simulink model "SIFT"  (R2016a)
settings: Solver=FixedStepDiscrete  SolverMode=SingleTasking  StartTime=0  StopTime=5  RelTol=1e-3
undefined symbols (not defined in the file): gray, Rec, SDTV
libraries: visionhdlfilter x4, hdlsllib x3, visionhdlio x2, visionconversions x1, visionsources x1, visiongeotforms x1
settings Model: Creator=Gururaja  LastModifiedBy=Gururaja
settings OptimizationCC: BlockReduction=off  ConditionallyExecuteInputs=off  DefaultParameterBehavior=Inlined
settings DebuggingCC: AlgebraicLoopMsg=error  SingleTaskRateTransMsg=error  ParameterPrecisionLossMsg=none  IntegerSaturationMsg=none
settings HardwareCC: ProdBitPerPointer=32  ProdLargestAtomicFloat=None  ProdIntDivRoundTo=Undefined  ProdEndianess=Unspecified  ProdWordSize=32  ProdHWDeviceType=ASIC/FPGA->ASIC/FPGA  ProdEqTarget=off

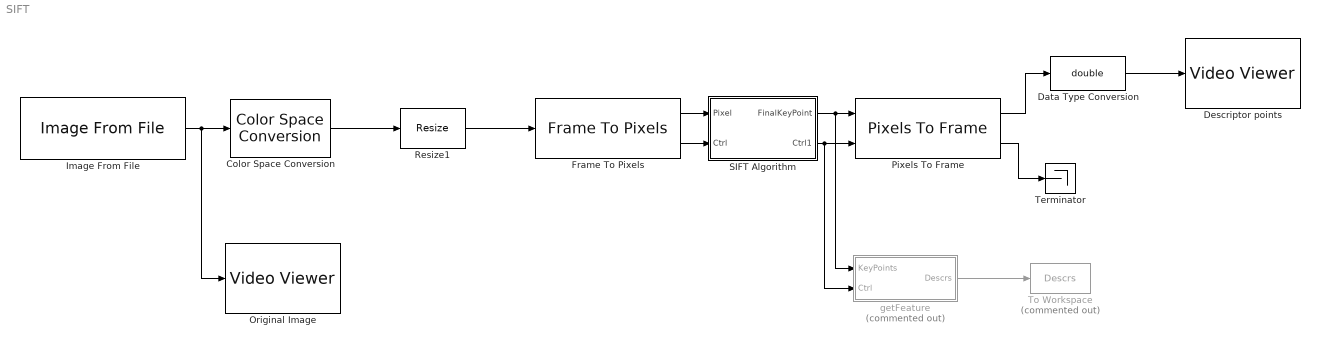
== system SIFT ==
  Color Space Conversion : visionconversions/Color Space  Conversion  conversion=Obsolete  conversionActive=R'G'B' to intensity  wp_str=D65  rec=Rec. 601 (SDTV)  sys=1125/60/2:1  imagePorts=One multidimensional signal
  Data Type Conversion : DataTypeConversion  OutDataTypeStr=double
  Descriptor points : VideoViewer  colormapValue=gray(256)  FigPos=[1 822 1536 724]
  Frame To Pixels : visionhdlio/Frame To Pixels  NumComponents=1  VideoFormat=240p  ActivePixelsPerLine=32  ActiveVideoLines=18  TotalPixelsPerLine=42  TotalVideoLines=28  StartingActiveLine=6  FrontPorch=5  SampleTime=0
  Image From File : visionsources/Image From File  Tag=vipblks_nd  FileName=E:\PROJECTS\FINAL YEAR PROJECT\ATTEMPTS\WORKING\SIFT-Scale-Invariant-Feature-Transform\lenatrain.jpg  imagePorts=One multidimensional signal  Ts=1  ImageDataType=Inherit from input image  Signed=off  WordLength=32  sdImageDataType=uint(8)  FractionLengthMode=Best precision  FractionLength=10  OutPortLabels=R|G|B
  Original Image : VideoViewer  colormapValue=gray(256)  FigPos=[1 822 1536 724]
  Pixels To Frame : visionhdlio/Pixels To Frame  NumComponents=1  VideoFormat=240p  ActivePixelsPerLine=32  ActiveVideoLines=18  TotalPixelsPerLine=42  TotalVideoLines=28
  Resize1 : visiongeotforms/Resize  specify=Number of output rows and columns  rfactor=[200 150]  outCols=25  outRows=25  outRowsCols=[240 320]  interp_method=Bilinear  antialias=on  useROI=off  roiFlag=off  prodOutputMode=Binary point scaling  prodOutputWordLength=32  prodOutputFracLength=10  roundingMode=Nearest  overflowMode=on
  SIFT Algorithm : Subsystem
  Terminator : Terminator
  To Workspace : ToWorkspace  Commented=on  VariableName=Descrs  SaveFormat=Timeseries  SampleTime=-1
  getFeature : Subsystem  Commented=on
  wires:
  Resize1/1 -> Frame To Pixels/1
  Frame To Pixels/1 -> SIFT Algorithm/1(Pixel)
  Frame To Pixels/2 -> SIFT Algorithm/2(Ctrl)
  SIFT Algorithm/1(FinalKeyPoint) -> getFeature/1(KeyPoints), Pixels To Frame/1
  SIFT Algorithm/2(Ctrl1) -> getFeature/2(Ctrl), Pixels To Frame/2
  Pixels To Frame/2 -> Terminator/1
  Pixels To Frame/1 -> Data Type Conversion/1
  Data Type Conversion/1 -> Descriptor points/1
  getFeature/1(Descrs) -> To Workspace/1
  Image From File/1 -> Original Image/1, Color Space Conversion/1
  Color Space Conversion/1 -> Resize1/1

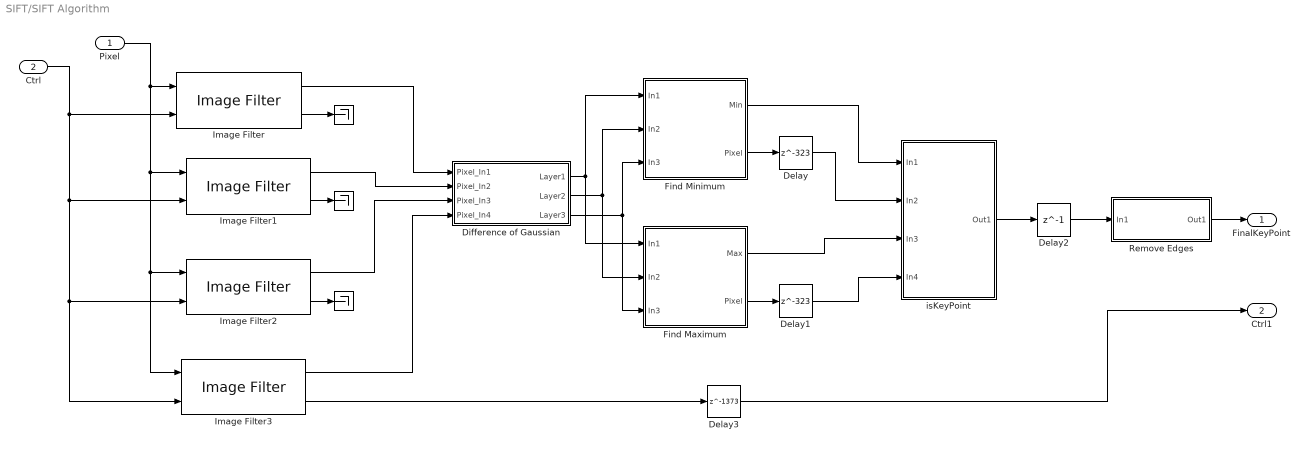
== system SIFT/SIFT Algorithm ==
  Pixel : Inport
  Ctrl : Inport  Port=2
  " " : Terminator
  " " : Terminator
  " " : Terminator
  Delay : Delay  DelayLength=323  InitialCondition=0
  Delay1 : Delay  DelayLength=323  InitialCondition=0
  Delay2 : Delay  DelayLength=1  InitialCondition=0
  Delay3 : Delay  DelayLength=1373  InitialCondition=0
  Difference of Gaussian : Subsystem
  Find Maximum : Subsystem
  Find Minimum : Subsystem
  Image Filter{,1..3} (4 alike) : visionhdlfilter/Image Filter  Coefficients=[ 1, 0; 0, -1 ]  PaddingMethod=Constant  PaddingValue=0  LineBufferSize=2048  roundingMode=Floor  overflowMode=off  CoeffMin=[]  CoeffMax=[]  OutputMin=[]  OutputMax=[]  SimulateUsing=Code generation
  Remove Edges : Subsystem
  isKeyPoint : Subsystem
  FinalKeyPoint : Outport
  Ctrl1 : Outport  Port=2
  wires:
  Pixel/1 -> Image Filter/1, Image Filter1/1, Image Filter3/1, Image Filter2/1
  Ctrl/1 -> Image Filter/2, Image Filter1/2, Image Filter2/2, Image Filter3/2
  Image Filter2/2 -> " "/1
  Image Filter1/2 -> " "/1
  Image Filter/2 -> " "/1
  Image Filter/1 -> Difference of Gaussian/1(Pixel_In1)
  Image Filter1/1 -> Difference of Gaussian/2(Pixel_In2)
  Image Filter2/1 -> Difference of Gaussian/3(Pixel_In3)
  Image Filter3/1 -> Difference of Gaussian/4(Pixel_In4)
  Difference of Gaussian/1(Layer1) -> Find Maximum/1(In1), Find Minimum/1(In1)
  Difference of Gaussian/2(Layer2) -> Find Maximum/2(In2), Find Minimum/2(In2)
  Difference of Gaussian/3(Layer3) -> Find Maximum/3(In3), Find Minimum/3(In3)
  Find Minimum/2(Pixel) -> Delay/1
  Find Minimum/1(Min) -> isKeyPoint/1(In1)
  Delay/1 -> isKeyPoint/2(In2)
  Delay1/1 -> isKeyPoint/4(In4)
  isKeyPoint/1(Out1) -> Delay2/1
  Delay2/1 -> Remove Edges/1(In1)
  Remove Edges/1(Out1) -> FinalKeyPoint/1
  Image Filter3/2 -> Delay3/1
  Delay3/1 -> Ctrl1/1
  Find Maximum/1(Max) -> isKeyPoint/3(In3)
  Find Maximum/2(Pixel) -> Delay1/1

== system SIFT/getFeature ==
  KeyPoints : Inport
  Ctrl : Inport  Port=2
  Delay : Delay  DelayLength=647  InitialCondition=0
  Delay1 : Delay  DelayLength=647  InitialCondition=0
  Descriptor : Subsystem
  HDL FIFO : hdlsllib/HDL Operations/HDL FIFO  fifo_size=1000  ratio=1  push_msg=Warning  pop_msg=Warning  show_empty=on  show_full=on  show_num=on
  MATLAB Function : MATLAB Function  TreatAsAtomicUnit=on
  MagORI : Subsystem
  Terminator : Terminator
  Terminator1 : Terminator
  Descrs : Outport
  wires:
  KeyPoints/1 -> HDL FIFO/1, Delay/1
  Delay/1 -> MagORI/1(Pixel)
  Ctrl/1 -> HDL FIFO/2, Delay1/1
  Delay1/1 -> MagORI/2(Ctrl)
  HDL FIFO/4 -> Terminator/1
  HDL FIFO/3 -> Terminator1/1
  MagORI/1(Mag) -> Descriptor/1(In1)
  HDL FIFO/2 -> MATLAB Function/3(empty)
  Descriptor/1(KeyPoint) -> MATLAB Function/2(KPdis)
  HDL FIFO/1 -> MATLAB Function/1(KPsource)
  Descriptor/2(Desc) -> MATLAB Function/4(descr)
  MATLAB Function/2(descrs) -> Descrs/1
  MATLAB Function/1(y) -> HDL FIFO/3

== system SIFT/SIFT Algorithm/Difference of Gaussian ==
  Pixel_In1 : Inport
  Pixel_In2 : Inport  Port=2
  Pixel_In3 : Inport  Port=3
  Pixel_In4 : Inport  Port=4
  Delay : Delay  DelayLength=13  InitialCondition=0
  Delay1 : Delay  DelayLength=1  InitialCondition=0
  Delay2 : Delay  DelayLength=1  InitialCondition=0
  Delay3 : Delay  DelayLength=12  InitialCondition=0
  Sum1 : Sum  Inputs=+-
  Sum2 : Sum  Inputs=+-
  Sum3 : Sum  Inputs=+-
  Layer1 : Outport
  Layer2 : Outport  Port=2
  Layer3 : Outport  Port=3
  wires:
  Pixel_In1/1 -> Sum3/1
  Pixel_In2/1 -> Sum3/2, Delay3/1
  Delay3/1 -> Sum1/1
  Pixel_In3/1 -> Sum2/1, Sum1/2
  Pixel_In4/1 -> Sum2/2
  Sum3/1 -> Delay/1
  Sum1/1 -> Delay1/1
  Sum2/1 -> Delay2/1
  Delay2/1 -> Layer3/1
  Delay1/1 -> Layer2/1
  Delay/1 -> Layer1/1

== system SIFT/SIFT Algorithm/Find Maximum ==
  In1 : Inport
  In2 : Inport  Port=2
  In3 : Inport  Port=3
  Min/Max DOG1 : Subsystem
  Min/Max DOG2 : Subsystem
  Min/Max DOG3 : Subsystem
  MinMax : MinMax  Function=max  Inputs=26
  Max : Outport
  Pixel : Outport  Port=2
  wires:
  In2/1 -> Min/Max DOG1/1(In1)
  Min/Max DOG1/5(Out5) -> Pixel/1
  Min/Max DOG2/1(Out1) -> MinMax/18
  Min/Max DOG2/9(Out9) -> MinMax/26
  Min/Max DOG2/2(Out2) -> MinMax/19
  Min/Max DOG2/3(Out3) -> MinMax/20
  Min/Max DOG2/4(Out4) -> MinMax/21
  Min/Max DOG2/5(Out5) -> MinMax/22
  Min/Max DOG2/6(Out6) -> MinMax/23
  Min/Max DOG2/7(Out7) -> MinMax/24
  Min/Max DOG2/8(Out8) -> MinMax/25
  Min/Max DOG3/1(Out1) -> MinMax/1
  Min/Max DOG3/3(Out3) -> MinMax/3
  Min/Max DOG3/2(Out2) -> MinMax/2
  Min/Max DOG3/4(Out4) -> MinMax/4
  Min/Max DOG3/5(Out5) -> MinMax/5
  Min/Max DOG3/6(Out6) -> MinMax/6
  Min/Max DOG3/7(Out7) -> MinMax/7
  Min/Max DOG3/8(Out8) -> MinMax/8
  Min/Max DOG3/9(Out9) -> MinMax/9
  MinMax/1 -> Max/1
  Min/Max DOG1/1(Out1) -> MinMax/10
  Min/Max DOG1/2(Out2) -> MinMax/11
  Min/Max DOG1/3(Out3) -> MinMax/12
  Min/Max DOG1/4(Out4) -> MinMax/13
  Min/Max DOG1/6(Out6) -> MinMax/14
  Min/Max DOG1/7(Out7) -> MinMax/15
  Min/Max DOG1/8(Out8) -> MinMax/16
  Min/Max DOG1/9(Out9) -> MinMax/17
  In1/1 -> Min/Max DOG3/1(In1)
  In3/1 -> Min/Max DOG2/1(In1)

== system SIFT/SIFT Algorithm/Find Minimum ==
  In1 : Inport
  In2 : Inport  Port=2
  In3 : Inport  Port=3
  Min/Max DOG1 : Subsystem
  Min/Max DOG2 : Subsystem
  Min/Max DOG3 : Subsystem
  MinMax : MinMax  Inputs=26
  Min : Outport
  Pixel : Outport  Port=2
  wires:
  In2/1 -> Min/Max DOG1/1(In1)
  Min/Max DOG1/5(Out5) -> Pixel/1
  Min/Max DOG2/1(Out1) -> MinMax/18
  Min/Max DOG2/9(Out9) -> MinMax/26
  Min/Max DOG2/2(Out2) -> MinMax/19
  Min/Max DOG2/3(Out3) -> MinMax/20
  Min/Max DOG2/4(Out4) -> MinMax/21
  Min/Max DOG2/5(Out5) -> MinMax/22
  Min/Max DOG2/6(Out6) -> MinMax/23
  Min/Max DOG2/7(Out7) -> MinMax/24
  Min/Max DOG2/8(Out8) -> MinMax/25
  Min/Max DOG3/1(Out1) -> MinMax/1
  Min/Max DOG3/3(Out3) -> MinMax/3
  Min/Max DOG3/2(Out2) -> MinMax/2
  Min/Max DOG3/4(Out4) -> MinMax/4
  Min/Max DOG3/5(Out5) -> MinMax/5
  Min/Max DOG3/6(Out6) -> MinMax/6
  Min/Max DOG3/7(Out7) -> MinMax/7
  Min/Max DOG3/8(Out8) -> MinMax/8
  Min/Max DOG3/9(Out9) -> MinMax/9
  MinMax/1 -> Min/1
  Min/Max DOG1/1(Out1) -> MinMax/10
  Min/Max DOG1/2(Out2) -> MinMax/11
  Min/Max DOG1/3(Out3) -> MinMax/12
  Min/Max DOG1/4(Out4) -> MinMax/13
  Min/Max DOG1/6(Out6) -> MinMax/14
  Min/Max DOG1/7(Out7) -> MinMax/15
  Min/Max DOG1/8(Out8) -> MinMax/16
  Min/Max DOG1/9(Out9) -> MinMax/17
  In1/1 -> Min/Max DOG3/1(In1)
  In3/1 -> Min/Max DOG2/1(In1)

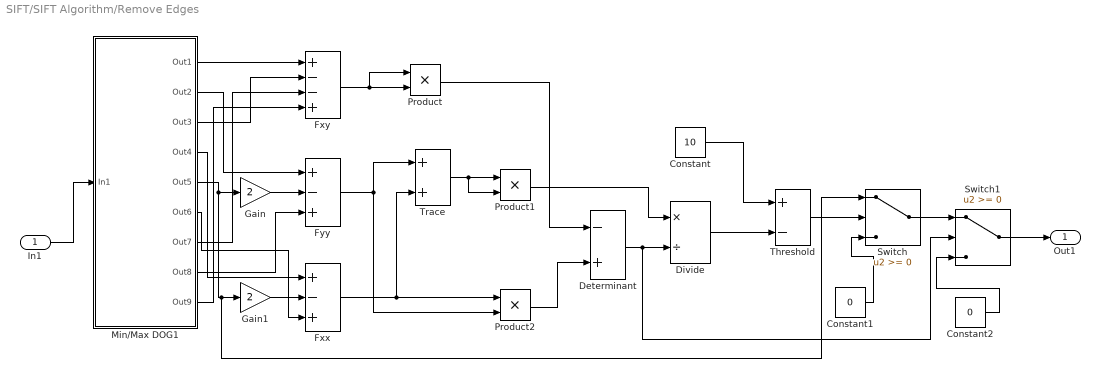
== system SIFT/SIFT Algorithm/Remove Edges ==
  In1 : Inport
  Constant : Constant  Value=10
  Constant1 : Constant  Value=0
  Constant2 : Constant  Value=0
  Determinant : Sum  Inputs=-+
  Divide : Product  Inputs=*/  SaturateOnIntegerOverflow=on
  Fxx : Sum  Inputs=+-+
  Fxy : Sum  Inputs=+--+
  Fyy : Sum  Inputs=+-+
  Gain : Gain  Gain=2
  Gain1 : Gain  Gain=2
  Min/Max DOG1 : Subsystem
  Product : Product
  Product1 : Product
  Product2 : Product
  Switch : Switch
  Switch1 : Switch
  Threshold : Sum  Inputs=+-
  Trace : Sum
  Out1 : Outport
  wires:
  In1/1 -> Min/Max DOG1/1(In1)
  Min/Max DOG1/1(Out1) -> Fxy/1
  Min/Max DOG1/3(Out3) -> Fxy/2
  Gain1/1 -> Fxx/2
  Gain/1 -> Fyy/2
  Min/Max DOG1/2(Out2) -> Fyy/1
  Min/Max DOG1/4(Out4) -> Fxx/1
  Min/Max DOG1/6(Out6) -> Fxx/3
  Min/Max DOG1/7(Out7) -> Fxy/3
  Min/Max DOG1/8(Out8) -> Fyy/3
  Min/Max DOG1/9(Out9) -> Fxy/4
  Fyy/1 -> Product2/2, Trace/1
  Fxy/1 -> Product/1, Product/2
  Trace/1 -> Product1/2, Product1/1
  Fxx/1 -> Trace/2, Product2/1
  Product2/1 -> Determinant/2
  Product/1 -> Determinant/1
  Determinant/1 -> Switch1/2, Divide/2
  Product1/1 -> Divide/1
  Divide/1 -> Threshold/2
  Constant/1 -> Threshold/1
  Threshold/1 -> Switch/2
  Constant1/1 -> Switch/3
  Min/Max DOG1/5(Out5) -> Switch/1, Gain1/1, Gain/1
  Switch/1 -> Switch1/1
  Constant2/1 -> Switch1/3
  Switch1/1 -> Out1/1

== system SIFT/SIFT Algorithm/isKeyPoint ==
  In1 : Inport
  In2 : Inport  Port=2
  In3 : Inport  Port=3
  In4 : Inport  Port=4
  " " : Constant  Value=0
  " " : Constant  Value=0
  Logical Operator : Logic  Operator=OR  AllPortsSameDT=off  OutDataTypeStr=boolean
  MinMax : MinMax  Function=max  Inputs=2
  Product : Product
  Product1 : Product
  Sum1 : Sum  Inputs=+-
  Sum2 : Sum  Inputs=+-
  Switch1 : Switch
  Switch2 : Switch
  Out1 : Outport
  wires:
  In1/1 -> Sum2/1
  In2/1 -> Sum2/2, Switch2/1, Product1/1
  Sum1/1 -> Switch1/2
  Sum2/1 -> Switch2/2
  " "/1 -> Switch2/3
  " "/1 -> Switch1/3
  In3/1 -> Sum1/1
  Switch2/1 -> Logical Operator/1
  Switch1/1 -> Logical Operator/2
  Product1/1 -> MinMax/1
  Product/1 -> MinMax/2
  MinMax/1 -> Out1/1
  Logical Operator/1 -> Product1/2, Product/1
  In4/1 -> Sum1/2, Switch1/1, Product/2

== system SIFT/getFeature/Descriptor ==
  In1 : Inport
  Delay : Delay  DelayLength=320  InitialCondition=0
  Delay1 : Delay  DelayLength=320  InitialCondition=0
  Delay2 : Delay  DelayLength=320  InitialCondition=0
  OriHist : Subsystem
  OriHist2 : Subsystem
  OriHist3 : Subsystem
  OriHistWithKey : Subsystem
  Reshape : MATLAB Function  TreatAsAtomicUnit=on
  KeyPoint : Outport
  Desc : Outport  Port=2
  wires:
  In1/1 -> OriHist/1(In1)
  Delay/1 -> OriHist3/1(In1)
  OriHist2/5(Out5) -> Delay/1
  Delay1/1 -> OriHist2/1(In1)
  OriHistWithKey/5(Out5) -> Delay1/1
  Delay2/1 -> OriHistWithKey/1(In1)
  OriHist/5(Out5) -> Delay2/1
  Reshape/1(y) -> Desc/1
  OriHistWithKey/6(KeyPoint) -> KeyPoint/1
  OriHist/1(Out1) -> Reshape/1(u1)
  OriHist/2(Out2) -> Reshape/2(u2)
  OriHist/3(Out3) -> Reshape/3(u3)
  OriHist/4(Out4) -> Reshape/4(u4)
  OriHistWithKey/1(Out1) -> Reshape/5(u5)
  OriHistWithKey/2(Out2) -> Reshape/6(u6)
  OriHistWithKey/3(Out3) -> Reshape/7(u7)
  OriHistWithKey/4(Out4) -> Reshape/8(u8)
  OriHist2/1(Out1) -> Reshape/9(u9)
  OriHist2/2(Out2) -> Reshape/10(u10)
  OriHist2/3(Out3) -> Reshape/11(u11)
  OriHist2/4(Out4) -> Reshape/12(u12)
  OriHist3/1(Out1) -> Reshape/13(u13)
  OriHist3/2(Out2) -> Reshape/14(u14)
  OriHist3/3(Out3) -> Reshape/15(u15)
  OriHist3/4(Out4) -> Reshape/16(u16)

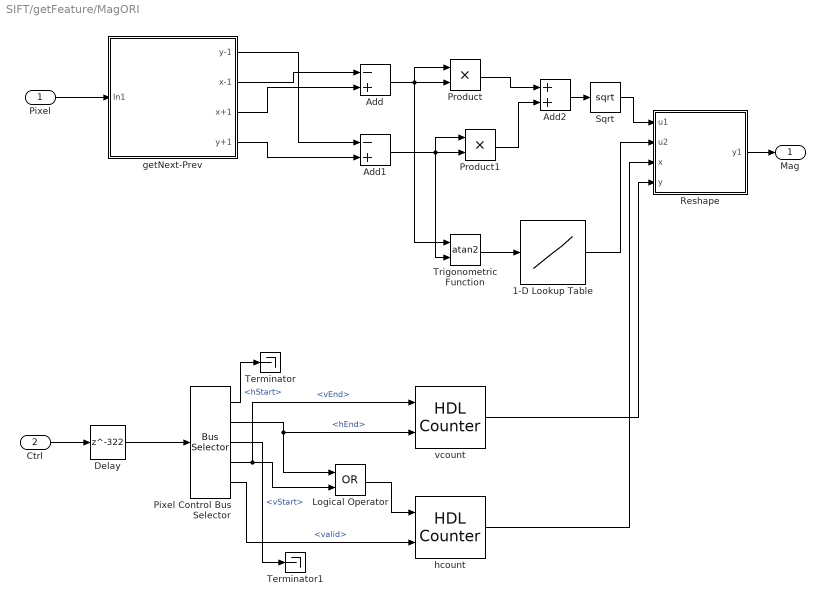
== system SIFT/getFeature/MagORI ==
  Pixel : Inport
  Ctrl : Inport  Port=2
  1-D Lookup Table : Lookup_n-D  NumberOfTableDimensions=1  BreakpointsForDimension1=[-5:5]  Table=tanh([-5:5])  InternalRulePriority=Speed  RndMeth=Simplest  InputSameDT=on
  Add : Sum  Inputs=-+
  Add1 : Sum  Inputs=-+
  Add2 : Sum
  Delay : Delay  DelayLength=322  InitialCondition=0
  Logical Operator : Logic  Operator=OR  AllPortsSameDT=off  OutDataTypeStr=boolean
  Pixel Control Bus Selector : BusSelector  OutputSignals=hStart,hEnd,vStart,vEnd,valid
  Product : Product
  Product1 : Product
  Reshape : MATLAB Function  TreatAsAtomicUnit=on
  Sqrt : Sqrt  SaturateOnIntegerOverflow=on
  Terminator : Terminator
  Terminator1 : Terminator
  Trigonometric Function : Trigonometry  Operator=atan2
  getNext-Prev : Subsystem
  hcount : hdlsllib/HDL Operations/HDL Counter  CountType=Count limited  CountInit=0  CountStep=1  CountMax=25  CountFromType=Initial value  CountFrom=0  CountResetPort=on  CountLoadPort=off  CountEnbPort=on  CountDirPort=off  CountDataType=Signed  CountWordLen=8  CountFracLen=0  CountSampTime=1
  vcount : hdlsllib/HDL Operations/HDL Counter  CountType=Count limited  CountInit=0  CountStep=1  CountMax=25  CountFromType=Initial value  CountFrom=0  CountResetPort=on  CountLoadPort=off  CountEnbPort=on  CountDirPort=off  CountDataType=Signed  CountWordLen=8  CountFracLen=0  CountSampTime=1
  Mag : Outport
  wires:
  Pixel/1 -> getNext-Prev/1(In1)
  getNext-Prev/1(y-1) -> Add1/1
  getNext-Prev/2(x-1) -> Add/1
  getNext-Prev/3(x+1) -> Add/2
  getNext-Prev/4(y+1) -> Add1/2
  Add/1 -> Trigonometric Function/1, Product/1, Product/2
  Add1/1 -> Trigonometric Function/2, Product1/1, Product1/2
  Product/1 -> Add2/1
  Product1/1 -> Add2/2
  Add2/1 -> Sqrt/1
  Reshape/1(y1) -> Mag/1
  Sqrt/1 -> Reshape/1(u1)
  Trigonometric Function/1 -> 1-D Lookup Table/1
  1-D Lookup Table/1 -> Reshape/2(u2)
  Ctrl/1 -> Delay/1
  Delay/1 -> Pixel Control Bus Selector/1
  Pixel Control Bus Selector/2 -> Logical Operator/1, vcount/2  "<hEnd>"
  Pixel Control Bus Selector/4 -> vcount/1, Logical Operator/2  "<vEnd>"
  Logical Operator/1 -> hcount/1
  Pixel Control Bus Selector/5 -> hcount/2  "<valid>"
  vcount/1 -> Reshape/4(y)
  hcount/1 -> Reshape/3(x)
  Pixel Control Bus Selector/1 -> Terminator/1  "<hStart>"
  Pixel Control Bus Selector/3 -> Terminator1/1  "<vStart>"

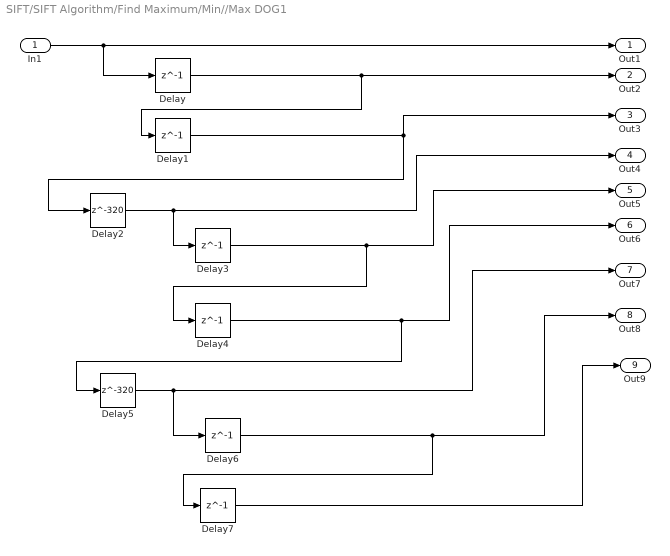
== system SIFT/SIFT Algorithm/Find Maximum/Min//Max DOG1 ==
  In1 : Inport
  Delay{,1,3..4,6..7} (6 alike) : Delay  DelayLength=1  InitialCondition=0
  Delay2 : Delay  DelayLength=320  InitialCondition=0
  Delay5 : Delay  DelayLength=320  InitialCondition=0
  Out1 : Outport
  Out2 : Outport  Port=2
  Out3 : Outport  Port=3
  Out4 : Outport  Port=4
  Out5 : Outport  Port=5
  Out6 : Outport  Port=6
  Out7 : Outport  Port=7
  Out8 : Outport  Port=8
  Out9 : Outport  Port=9
  wires:
  In1/1 -> Delay/1, Out1/1
  Delay/1 -> Out2/1, Delay1/1
  Delay1/1 -> Out3/1, Delay2/1
  Delay2/1 -> Delay3/1, Out4/1
  Delay3/1 -> Delay4/1, Out5/1
  Delay4/1 -> Delay5/1, Out6/1
  Delay5/1 -> Delay6/1, Out7/1
  Delay6/1 -> Delay7/1, Out8/1
  Delay7/1 -> Out9/1

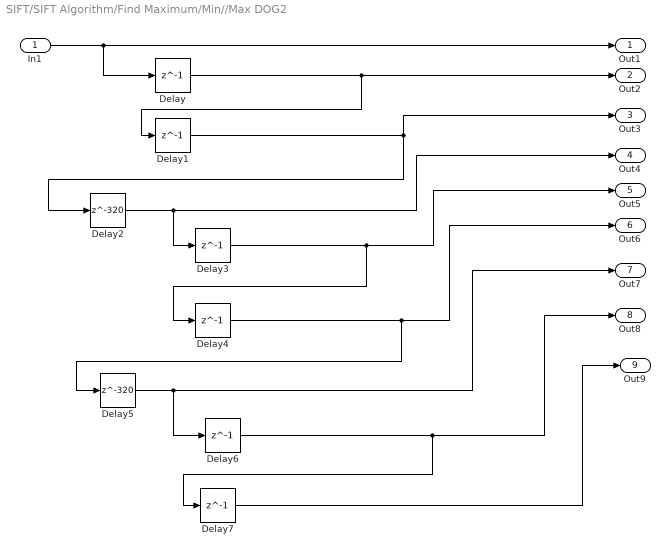
== system SIFT/SIFT Algorithm/Find Maximum/Min//Max DOG2 ==
  In1 : Inport
  Delay{,1,3..4,6..7} (6 alike) : Delay  DelayLength=1  InitialCondition=0
  Delay2 : Delay  DelayLength=320  InitialCondition=0
  Delay5 : Delay  DelayLength=320  InitialCondition=0
  Out1 : Outport
  Out2 : Outport  Port=2
  Out3 : Outport  Port=3
  Out4 : Outport  Port=4
  Out5 : Outport  Port=5
  Out6 : Outport  Port=6
  Out7 : Outport  Port=7
  Out8 : Outport  Port=8
  Out9 : Outport  Port=9
  wires:
  In1/1 -> Delay/1, Out1/1
  Delay/1 -> Out2/1, Delay1/1
  Delay1/1 -> Out3/1, Delay2/1
  Delay2/1 -> Delay3/1, Out4/1
  Delay3/1 -> Delay4/1, Out5/1
  Delay4/1 -> Delay5/1, Out6/1
  Delay5/1 -> Delay6/1, Out7/1
  Delay6/1 -> Delay7/1, Out8/1
  Delay7/1 -> Out9/1

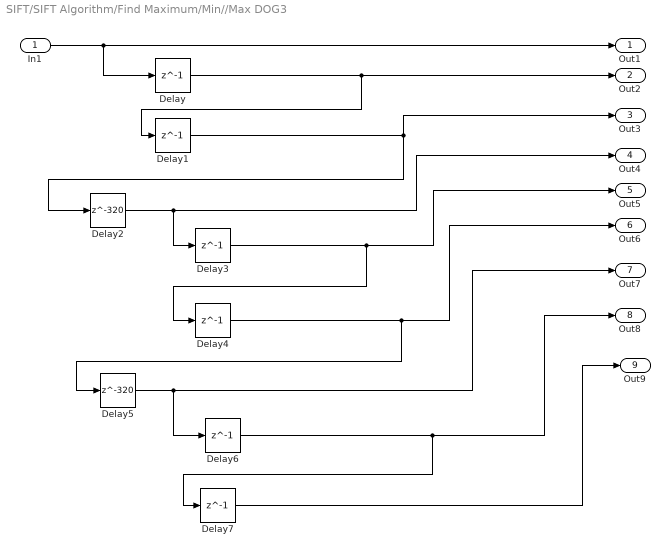
== system SIFT/SIFT Algorithm/Find Maximum/Min//Max DOG3 ==
  In1 : Inport
  Delay{,1,3..4,6..7} (6 alike) : Delay  DelayLength=1  InitialCondition=0
  Delay2 : Delay  DelayLength=320  InitialCondition=0
  Delay5 : Delay  DelayLength=320  InitialCondition=0
  Out1 : Outport
  Out2 : Outport  Port=2
  Out3 : Outport  Port=3
  Out4 : Outport  Port=4
  Out5 : Outport  Port=5
  Out6 : Outport  Port=6
  Out7 : Outport  Port=7
  Out8 : Outport  Port=8
  Out9 : Outport  Port=9
  wires:
  In1/1 -> Delay/1, Out1/1
  Delay/1 -> Out2/1, Delay1/1
  Delay1/1 -> Out3/1, Delay2/1
  Delay2/1 -> Delay3/1, Out4/1
  Delay3/1 -> Delay4/1, Out5/1
  Delay4/1 -> Delay5/1, Out6/1
  Delay5/1 -> Delay6/1, Out7/1
  Delay6/1 -> Delay7/1, Out8/1
  Delay7/1 -> Out9/1

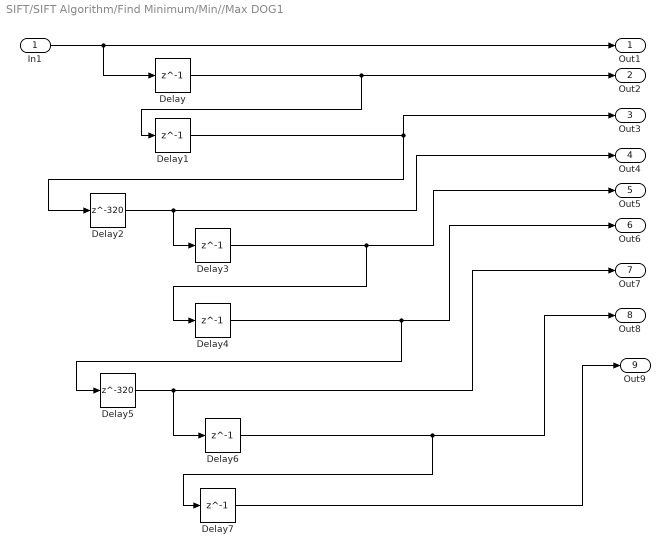
== system SIFT/SIFT Algorithm/Find Minimum/Min//Max DOG1 ==
  In1 : Inport
  Delay{,1,3..4,6..7} (6 alike) : Delay  DelayLength=1  InitialCondition=0
  Delay2 : Delay  DelayLength=320  InitialCondition=0
  Delay5 : Delay  DelayLength=320  InitialCondition=0
  Out1 : Outport
  Out2 : Outport  Port=2
  Out3 : Outport  Port=3
  Out4 : Outport  Port=4
  Out5 : Outport  Port=5
  Out6 : Outport  Port=6
  Out7 : Outport  Port=7
  Out8 : Outport  Port=8
  Out9 : Outport  Port=9
  wires:
  In1/1 -> Delay/1, Out1/1
  Delay/1 -> Out2/1, Delay1/1
  Delay1/1 -> Out3/1, Delay2/1
  Delay2/1 -> Delay3/1, Out4/1
  Delay3/1 -> Delay4/1, Out5/1
  Delay4/1 -> Delay5/1, Out6/1
  Delay5/1 -> Delay6/1, Out7/1
  Delay6/1 -> Delay7/1, Out8/1
  Delay7/1 -> Out9/1

== system SIFT/SIFT Algorithm/Find Minimum/Min//Max DOG2 ==
  In1 : Inport
  Delay{,1,3..4,6..7} (6 alike) : Delay  DelayLength=1  InitialCondition=0
  Delay2 : Delay  DelayLength=320  InitialCondition=0
  Delay5 : Delay  DelayLength=320  InitialCondition=0
  Out1 : Outport
  Out2 : Outport  Port=2
  Out3 : Outport  Port=3
  Out4 : Outport  Port=4
  Out5 : Outport  Port=5
  Out6 : Outport  Port=6
  Out7 : Outport  Port=7
  Out8 : Outport  Port=8
  Out9 : Outport  Port=9
  wires:
  In1/1 -> Delay/1, Out1/1
  Delay/1 -> Out2/1, Delay1/1
  Delay1/1 -> Out3/1, Delay2/1
  Delay2/1 -> Delay3/1, Out4/1
  Delay3/1 -> Delay4/1, Out5/1
  Delay4/1 -> Delay5/1, Out6/1
  Delay5/1 -> Delay6/1, Out7/1
  Delay6/1 -> Delay7/1, Out8/1
  Delay7/1 -> Out9/1

== system SIFT/SIFT Algorithm/Find Minimum/Min//Max DOG3 ==
  In1 : Inport
  Delay{,1,3..4,6..7} (6 alike) : Delay  DelayLength=1  InitialCondition=0
  Delay2 : Delay  DelayLength=320  InitialCondition=0
  Delay5 : Delay  DelayLength=320  InitialCondition=0
  Out1 : Outport
  Out2 : Outport  Port=2
  Out3 : Outport  Port=3
  Out4 : Outport  Port=4
  Out5 : Outport  Port=5
  Out6 : Outport  Port=6
  Out7 : Outport  Port=7
  Out8 : Outport  Port=8
  Out9 : Outport  Port=9
  wires:
  In1/1 -> Delay/1, Out1/1
  Delay/1 -> Out2/1, Delay1/1
  Delay1/1 -> Out3/1, Delay2/1
  Delay2/1 -> Delay3/1, Out4/1
  Delay3/1 -> Delay4/1, Out5/1
  Delay4/1 -> Delay5/1, Out6/1
  Delay5/1 -> Delay6/1, Out7/1
  Delay6/1 -> Delay7/1, Out8/1
  Delay7/1 -> Out9/1

== system SIFT/SIFT Algorithm/Remove Edges/Min//Max DOG1 ==
  In1 : Inport
  Delay{,1,3..4,6..7} (6 alike) : Delay  DelayLength=1  InitialCondition=0
  Delay2 : Delay  DelayLength=320  InitialCondition=0
  Delay5 : Delay  DelayLength=320  InitialCondition=0
  Out1 : Outport
  Out2 : Outport  Port=2
  Out3 : Outport  Port=3
  Out4 : Outport  Port=4
  Out5 : Outport  Port=5
  Out6 : Outport  Port=6
  Out7 : Outport  Port=7
  Out8 : Outport  Port=8
  Out9 : Outport  Port=9
  wires:
  In1/1 -> Delay/1, Out1/1
  Delay/1 -> Out2/1, Delay1/1
  Delay1/1 -> Out3/1, Delay2/1
  Delay2/1 -> Delay3/1, Out4/1
  Delay3/1 -> Delay4/1, Out5/1
  Delay4/1 -> Delay5/1, Out6/1
  Delay5/1 -> Delay6/1, Out7/1
  Delay6/1 -> Delay7/1, Out8/1
  Delay7/1 -> Out9/1

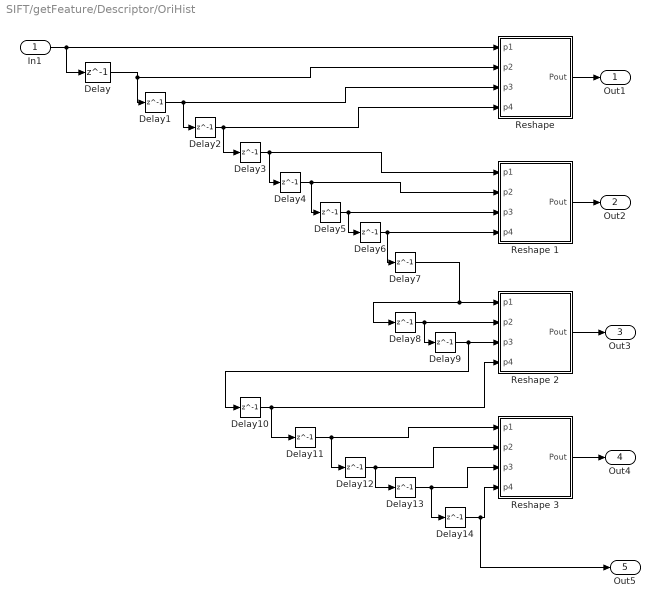
== system SIFT/getFeature/Descriptor/OriHist ==
  In1 : Inport
  Delay{,1..14} (15 alike) : Delay  DelayLength=1  InitialCondition=0
  "Reshape " : MATLAB Function  TreatAsAtomicUnit=on
  Reshape 1 : MATLAB Function  TreatAsAtomicUnit=on
  Reshape 2 : MATLAB Function  TreatAsAtomicUnit=on
  Reshape 3 : MATLAB Function  TreatAsAtomicUnit=on
  Out1 : Outport
  Out2 : Outport  Port=2
  Out3 : Outport  Port=3
  Out4 : Outport  Port=4
  Out5 : Outport  Port=5
  wires:
  "Reshape "/1(Pout) -> Out1/1
  Reshape 1/1(Pout) -> Out2/1
  Reshape 2/1(Pout) -> Out3/1
  Reshape 3/1(Pout) -> Out4/1
  In1/1 -> Delay/1, "Reshape "/1(p1)
  Delay/1 -> "Reshape "/2(p2), Delay1/1
  Delay1/1 -> Delay2/1, "Reshape "/3(p3)
  Delay2/1 -> Delay3/1, "Reshape "/4(p4)
  Delay3/1 -> Delay4/1, Reshape 1/1(p1)
  Delay4/1 -> Delay5/1, Reshape 1/2(p2)
  Delay5/1 -> Delay6/1, Reshape 1/3(p3)
  Delay6/1 -> Delay7/1, Reshape 1/4(p4)
  Delay7/1 -> Delay8/1, Reshape 2/1(p1)
  Delay8/1 -> Delay9/1, Reshape 2/2(p2)
  Delay9/1 -> Delay10/1, Reshape 2/3(p3)
  Delay10/1 -> Delay11/1, Reshape 2/4(p4)
  Delay11/1 -> Delay12/1, Reshape 3/1(p1)
  Delay12/1 -> Delay13/1, Reshape 3/2(p2)
  Delay13/1 -> Delay14/1, Reshape 3/3(p3)
  Delay14/1 -> Out5/1, Reshape 3/4(p4)

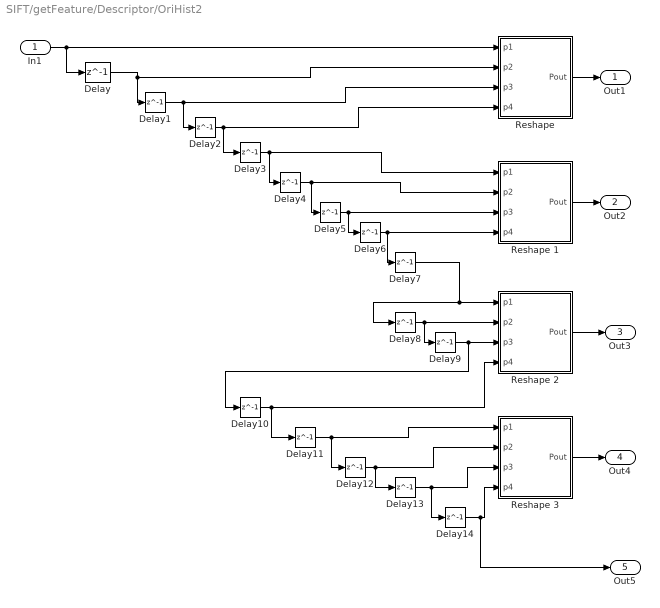
== system SIFT/getFeature/Descriptor/OriHist2 ==
  In1 : Inport
  Delay{,1..14} (15 alike) : Delay  DelayLength=1  InitialCondition=0
  "Reshape " : MATLAB Function  TreatAsAtomicUnit=on
  Reshape 1 : MATLAB Function  TreatAsAtomicUnit=on
  Reshape 2 : MATLAB Function  TreatAsAtomicUnit=on
  Reshape 3 : MATLAB Function  TreatAsAtomicUnit=on
  Out1 : Outport
  Out2 : Outport  Port=2
  Out3 : Outport  Port=3
  Out4 : Outport  Port=4
  Out5 : Outport  Port=5
  wires:
  "Reshape "/1(Pout) -> Out1/1
  Reshape 1/1(Pout) -> Out2/1
  Reshape 2/1(Pout) -> Out3/1
  Reshape 3/1(Pout) -> Out4/1
  In1/1 -> Delay/1, "Reshape "/1(p1)
  Delay/1 -> "Reshape "/2(p2), Delay1/1
  Delay1/1 -> Delay2/1, "Reshape "/3(p3)
  Delay2/1 -> Delay3/1, "Reshape "/4(p4)
  Delay3/1 -> Delay4/1, Reshape 1/1(p1)
  Delay4/1 -> Delay5/1, Reshape 1/2(p2)
  Delay5/1 -> Delay6/1, Reshape 1/3(p3)
  Delay6/1 -> Delay7/1, Reshape 1/4(p4)
  Delay7/1 -> Delay8/1, Reshape 2/1(p1)
  Delay8/1 -> Delay9/1, Reshape 2/2(p2)
  Delay9/1 -> Delay10/1, Reshape 2/3(p3)
  Delay10/1 -> Delay11/1, Reshape 2/4(p4)
  Delay11/1 -> Delay12/1, Reshape 3/1(p1)
  Delay12/1 -> Delay13/1, Reshape 3/2(p2)
  Delay13/1 -> Delay14/1, Reshape 3/3(p3)
  Delay14/1 -> Out5/1, Reshape 3/4(p4)

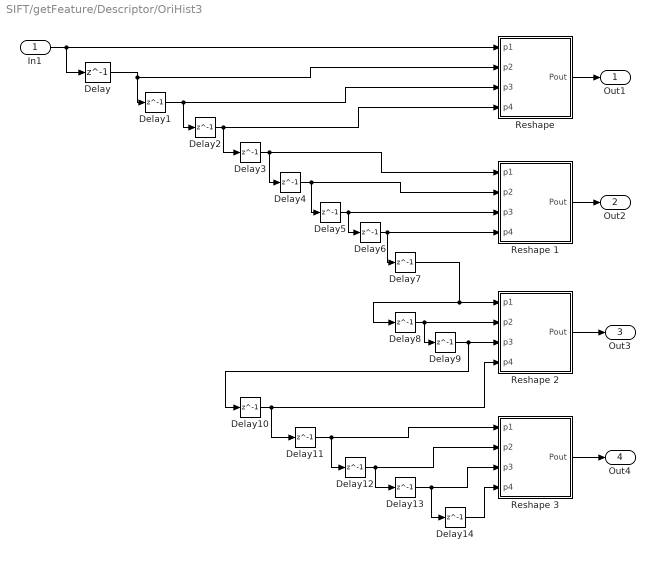
== system SIFT/getFeature/Descriptor/OriHist3 ==
  In1 : Inport
  Delay{,1..14} (15 alike) : Delay  DelayLength=1  InitialCondition=0
  "Reshape " : MATLAB Function  TreatAsAtomicUnit=on
  Reshape 1 : MATLAB Function  TreatAsAtomicUnit=on
  Reshape 2 : MATLAB Function  TreatAsAtomicUnit=on
  Reshape 3 : MATLAB Function  TreatAsAtomicUnit=on
  Out1 : Outport
  Out2 : Outport  Port=2
  Out3 : Outport  Port=3
  Out4 : Outport  Port=4
  wires:
  "Reshape "/1(Pout) -> Out1/1
  Reshape 1/1(Pout) -> Out2/1
  Reshape 2/1(Pout) -> Out3/1
  Reshape 3/1(Pout) -> Out4/1
  In1/1 -> Delay/1, "Reshape "/1(p1)
  Delay/1 -> "Reshape "/2(p2), Delay1/1
  Delay1/1 -> Delay2/1, "Reshape "/3(p3)
  Delay2/1 -> Delay3/1, "Reshape "/4(p4)
  Delay3/1 -> Delay4/1, Reshape 1/1(p1)
  Delay4/1 -> Delay5/1, Reshape 1/2(p2)
  Delay5/1 -> Delay6/1, Reshape 1/3(p3)
  Delay6/1 -> Delay7/1, Reshape 1/4(p4)
  Delay7/1 -> Delay8/1, Reshape 2/1(p1)
  Delay8/1 -> Delay9/1, Reshape 2/2(p2)
  Delay9/1 -> Delay10/1, Reshape 2/3(p3)
  Delay10/1 -> Delay11/1, Reshape 2/4(p4)
  Delay11/1 -> Delay12/1, Reshape 3/1(p1)
  Delay12/1 -> Delay13/1, Reshape 3/2(p2)
  Delay13/1 -> Delay14/1, Reshape 3/3(p3)
  Delay14/1 -> Reshape 3/4(p4)

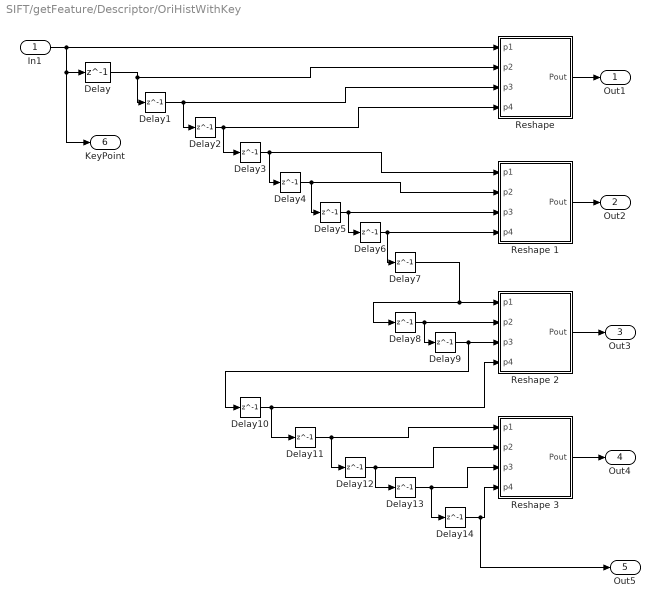
== system SIFT/getFeature/Descriptor/OriHistWithKey ==
  In1 : Inport
  Delay{,1..14} (15 alike) : Delay  DelayLength=1  InitialCondition=0
  "Reshape " : MATLAB Function  TreatAsAtomicUnit=on
  Reshape 1 : MATLAB Function  TreatAsAtomicUnit=on
  Reshape 2 : MATLAB Function  TreatAsAtomicUnit=on
  Reshape 3 : MATLAB Function  TreatAsAtomicUnit=on
  Out1 : Outport
  Out2 : Outport  Port=2
  Out3 : Outport  Port=3
  Out4 : Outport  Port=4
  Out5 : Outport  Port=5
  KeyPoint : Outport  Port=6
  wires:
  "Reshape "/1(Pout) -> Out1/1
  Reshape 1/1(Pout) -> Out2/1
  Reshape 2/1(Pout) -> Out3/1
  Reshape 3/1(Pout) -> Out4/1
  In1/1 -> KeyPoint/1, Delay/1, "Reshape "/1(p1)
  Delay/1 -> "Reshape "/2(p2), Delay1/1
  Delay1/1 -> Delay2/1, "Reshape "/3(p3)
  Delay2/1 -> Delay3/1, "Reshape "/4(p4)
  Delay3/1 -> Delay4/1, Reshape 1/1(p1)
  Delay4/1 -> Delay5/1, Reshape 1/2(p2)
  Delay5/1 -> Delay6/1, Reshape 1/3(p3)
  Delay6/1 -> Delay7/1, Reshape 1/4(p4)
  Delay7/1 -> Delay8/1, Reshape 2/1(p1)
  Delay8/1 -> Delay9/1, Reshape 2/2(p2)
  Delay9/1 -> Delay10/1, Reshape 2/3(p3)
  Delay10/1 -> Delay11/1, Reshape 2/4(p4)
  Delay11/1 -> Delay12/1, Reshape 3/1(p1)
  Delay12/1 -> Delay13/1, Reshape 3/2(p2)
  Delay13/1 -> Delay14/1, Reshape 3/3(p3)
  Delay14/1 -> Out5/1, Reshape 3/4(p4)

== system SIFT/getFeature/MagORI/getNext-Prev ==
  In1 : Inport
  Constant : Constant
  Constant1 : Constant
  Demux : Demux  Outputs=2
  Sum : Sum  Inputs=|++
  Sum1 : Sum  Inputs=|+-
  Sum2 : Sum  Inputs=|++
  Sum3 : Sum  Inputs=|+-
  y-1 : Outport
  x-1 : Outport  Port=2
  x+1 : Outport  Port=3
  y+1 : Outport  Port=4
  wires:
  In1/1 -> Demux/1
  Demux/1 -> Sum1/1, Sum/1
  Constant/1 -> Sum1/2, Sum/2
  Sum/1 -> x+1/1
  Sum1/1 -> x-1/1
  Demux/2 -> Sum2/1, Sum3/1
  Constant1/1 -> Sum3/2, Sum2/2
  Sum2/1 -> y+1/1
  Sum3/1 -> y-1/1

== matlab function SIFT/getFeature/MagORI/Reshape ==
  data: u1 input; y1 output; u2 input; x input; y input
function y1  = fcn(u1,u2,x,y)
%#codegen
y1 = [u1, u2, y, x];
end

== matlab function SIFT/getFeature/MATLAB Function ==
  data: KPsource input; y output; KPdis input; empty input; descr input; descrs output
function [y, descrs] = fcn(KPsource, KPdis, empty, descr)
%#codegen
descrs = descr;
y = 10;
end

== matlab function SIFT/getFeature/Descriptor/OriHist/Reshape  ==
  data: p1 input; Pout output; p2 input; p3 input; p4 input
function Pout = fcn(p1,p2,p3,p4)
%#codegen
pout = p1 + p2 + p3 + p4;
end

== matlab function SIFT/getFeature/Descriptor/OriHist/Reshape 1 ==
  data: p1 input; Pout output; p2 input; p3 input; p4 input
function Pout = fcn(p1,p2,p3,p4)
%#codegen
pout = p1 + p2 + p3 + p4;
end

== matlab function SIFT/getFeature/Descriptor/OriHist/Reshape 2 ==
  data: p1 input; Pout output; p2 input; p3 input; p4 input
function Pout = fcn(p1,p2,p3,p4)
%#codegen
pout = p1 + p2 + p3 + p4;
end

== matlab function SIFT/getFeature/Descriptor/OriHist/Reshape 3 ==
  data: p1 input; Pout output; p2 input; p3 input; p4 input
function Pout = fcn(p1,p2,p3,p4)
%#codegen
pout = p1 + p2 + p3 + p4;
end

== matlab function SIFT/getFeature/Descriptor/OriHistWithKey/Reshape  ==
  data: p1 input; Pout output; p2 input; p3 input; p4 input
function Pout = fcn(p1,p2,p3,p4)
%#codegen
pout = p1 + p2 + p3 + p4;
end

== matlab function SIFT/getFeature/Descriptor/OriHistWithKey/Reshape 1 ==
  data: p1 input; Pout output; p2 input; p3 input; p4 input
function Pout = fcn(p1,p2,p3,p4)
%#codegen
pout = p1 + p2 + p3 + p4;
end

== matlab function SIFT/getFeature/Descriptor/OriHistWithKey/Reshape 2 ==
  data: p1 input; Pout output; p2 input; p3 input; p4 input
function Pout = fcn(p1,p2,p3,p4)
%#codegen

pout = p1 + p2 + p3 + p4;
end

== matlab function SIFT/getFeature/Descriptor/OriHistWithKey/Reshape 3 ==
  data: p1 input; Pout output; p2 input; p3 input; p4 input
function Pout = fcn(p1,p2,p3,p4)
%#codegen

pout = p1 + p2 + p3 + p4;
end

== matlab function SIFT/getFeature/Descriptor/OriHist2/Reshape  ==
  data: p1 input; Pout output; p2 input; p3 input; p4 input
function Pout = fcn(p1,p2,p3,p4)
%#codegen

pout = p1 + p2 + p3 + p4;
end

== matlab function SIFT/getFeature/Descriptor/OriHist2/Reshape 1 ==
  data: p1 input; Pout output; p2 input; p3 input; p4 input
function Pout = fcn(p1,p2,p3,p4)
%#codegen

pout = p1 + p2 + p3 + p4;
end

== matlab function SIFT/getFeature/Descriptor/OriHist2/Reshape 2 ==
  data: p1 input; Pout output; p2 input; p3 input; p4 input
function Pout = fcn(p1,p2,p3,p4)
%#codegen

pout = p1 + p2 + p3 + p4;
end

== matlab function SIFT/getFeature/Descriptor/OriHist2/Reshape 3 ==
  data: p1 input; Pout output; p2 input; p3 input; p4 input
function Pout = fcn(p1,p2,p3,p4)
%#codegen

pout = p1 + p2 + p3 + p4;
end

== matlab function SIFT/getFeature/Descriptor/OriHist3/Reshape  ==
  data: p1 input; Pout output; p2 input; p3 input; p4 input
function Pout = fcn(p1,p2,p3,p4)
%#codegen

pout = p1 + p2 + p3 + p4;
end

== matlab function SIFT/getFeature/Descriptor/OriHist3/Reshape 1 ==
  data: p1 input; Pout output; p2 input; p3 input; p4 input
function Pout = fcn(p1,p2,p3,p4)
%#codegen

pout = p1 + p2 + p3 + p4;
end

== matlab function SIFT/getFeature/Descriptor/OriHist3/Reshape 2 ==
  data: p1 input; Pout output; p2 input; p3 input; p4 input
function Pout = fcn(p1,p2,p3,p4)
%#codegen

pout = p1 + p2 + p3 + p4;
end

== matlab function SIFT/getFeature/Descriptor/OriHist3/Reshape 3 ==
  data: p1 input; Pout output; p2 input; p3 input; p4 input
function Pout = fcn(p1,p2,p3,p4)
%#codegen

pout = p1 + p2 + p3 + p4;
end

== matlab function SIFT/getFeature/Descriptor/Reshape ==
  data: u1 input; y output; u2 input; u3 input; u4 input; u5 input; u6 input; u7 input; u8 input; u9 input; u10 input; u11 input; u12 input; u13 input; u14 input; u15 input; u16 input
function y = fcn(u1,u2,u3,u4,u5,u6,u7,u8,u9,u10,u11,u12,u13,u14,u15,u16)
%#codegen
y = [u1, u2, u3, u4, u5, u6, u7, u8, u9, u10, u11, u12, u13, u14, u15, u16];
end
